simulink model "Lab2_Challenge"  (R2020b)
settings: Solver=VariableStepAuto  StartTime=0.0  StopTime=Time_of_simulation  RelTol=1e-3
undefined symbols (not defined in the file): A0, B0, Beq_hat, C, C0, D0, D_H_1, daq, degs2rpm, DiscIntNeverNeededParam, drv, Gamma_o, gbox, H, H_o, J_o, Jeq, K, K_I, Kw, Kw2, mot, N_H_1, Nr, Nu, Nx, Phi_o, rads2rpm, rpm2rads, sens, Step_ref, T, Ts
settings Model: Creator=Davide  LastModifiedBy=Musta

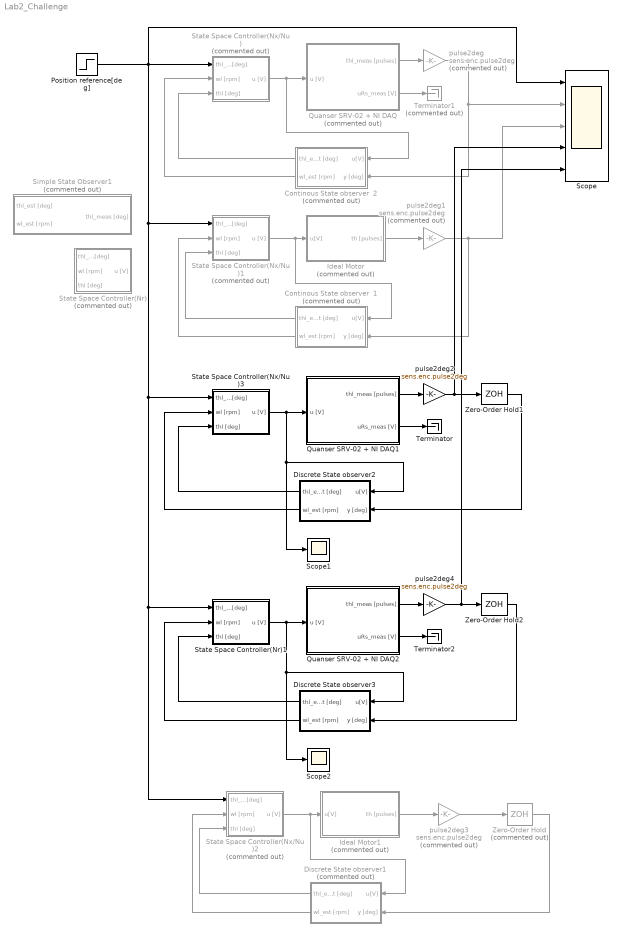
== system Lab2_Challenge ==
  Continous State observer  1 : Subsystem  Commented=on
  Continous State observer  2 : Subsystem  Commented=on
  Discrete State observer1 : Subsystem  Commented=on
  Discrete State observer2 : Subsystem
  Discrete State observer3 : Subsystem
  Ideal Motor : Subsystem  Commented=on
  Ideal Motor1 : Subsystem  Commented=on
  Position reference[deg] : Step  Time=0  After=Step_ref  SampleTime=0
  Quanser SRV-02 + NI DAQ : Subsystem  Commented=on  mask(Quanser SRV-02 (with inertial load) + NI DAQ){Ts=0.001, fricType=Coulomb + viscous}
      mask prompts: Ts "NI DAQ Sample Time:"; fricType "Friction model"
      mask help: Quanser SRV-02 (with inertial load) + NI DAQ model.
      mask init:
      | %%  Sensors data
      | 
      | %   shunt resistor
      | sens.curr.Rs = 0.5;                         %   resistance [Ohm]   
      | sens.curr.uRs_std = 0.01;                   %   voltage noise standard dev [V]                           
      | sens.curr.uRs_var = sens.curr.uRs_std^2;	%   voltage noise variance [V^2]
      | 
      | %   Hewlett-Packard HEDS-5540#A06 optical encoder
      | sens.enc.ppr = 500*4;                       %   pulses per rotation
      | sens.enc.pulse2deg = 360/sens.enc.ppr;      %   [pulses] -> [deg]
      | sens.enc.pulse2rad = 2*pi/sens.enc.ppr;     %   [pulses] -> [rad]
      | sens.enc.deg2pulse = sens.enc.ppr/360;      %   [deg] -> [pulses]
      | sens.enc.rad2pulse = sens.enc.ppr/2/pi;     %   [rad] -> [pulses]
      | 
      | 
      | %%  Data acquisition board (daq) data
      | 
      | %   NI PCI-6221 DAC data
      | daq.dac.bits = 16;                                  %   resolution (bits)
      | daq.dac.fs   = 10;                                  %   full scale 
      | daq.dac.q    = 2*daq.dac.fs/(2^daq.dac.bits-1);     %	quantization
      | 
      | %   NI PCI-6221 ADC data
      | daq.adc.bits = 16;                                  %   resolution (bits)
      | daq.adc.fs   = 10;                                  %   full scale (as set in SLDRT Analog Input block)
      | daq.adc.q    = 2*daq.adc.fs/(2^daq.adc.bits-1);     %   quantization
      mask Help:
      | Riccardo Antonello (antonello@dei.unipd.it)
      | 
      | April 24, 2020
      | 
      | Dept. of Information Engineering, University of Padova
      mask TypeOptions fricType: Coulomb + viscous | Karnopp
  Quanser SRV-02 + NI DAQ1 : Subsystem  mask(Quanser SRV-02 (with inertial load) + NI DAQ){Ts=T, fricType=Karnopp}
      mask prompts: Ts "NI DAQ Sample Time:"; fricType "Friction model"
      mask help: Quanser SRV-02 (with inertial load) + NI DAQ model.
      mask init: same as Lab2_Challenge/Quanser SRV-02 + NI DAQ
      mask Help:
      | Riccardo Antonello (antonello@dei.unipd.it)
      | 
      | April 24, 2020
      | 
      | Dept. of Information Engineering, University of Padova
      mask TypeOptions fricType: Coulomb + viscous | Karnopp
  Quanser SRV-02 + NI DAQ2 : Subsystem  mask(Quanser SRV-02 (with inertial load) + NI DAQ){Ts=T, fricType=Karnopp}
      mask prompts: Ts "NI DAQ Sample Time:"; fricType "Friction model"
      mask help: Quanser SRV-02 (with inertial load) + NI DAQ model.
      mask init: same as Lab2_Challenge/Quanser SRV-02 + NI DAQ
      mask Help:
      | Riccardo Antonello (antonello@dei.unipd.it)
      | 
      | April 24, 2020
      | 
      | Dept. of Information Engineering, University of Padova
      mask TypeOptions fricType: Coulomb + viscous | Karnopp
  Scope : Scope  NumInputPorts=5
  Scope1 : Scope
  Scope2 : Scope
  Simple State Observer1 : Subsystem  Commented=on
  State Space Controller(Nr) : Subsystem  Commented=on
  State Space Controller(Nr)1 : Subsystem
  State Space Controller(Nx/Nu) : Subsystem  Commented=on
  State Space Controller(Nx/Nu)1 : Subsystem  Commented=on
  State Space Controller(Nx/Nu)2 : Subsystem  Commented=on
  State Space Controller(Nx/Nu)3 : Subsystem
  Terminator : Terminator
  Terminator1 : Terminator  Commented=on
  Terminator2 : Terminator
  Zero-Order Hold : ZeroOrderHold  Commented=on  SampleTime=T
  Zero-Order Hold1 : ZeroOrderHold  SampleTime=T
  Zero-Order Hold2 : ZeroOrderHold  SampleTime=T
  pulse2deg : Gain  Commented=on  Gain=sens.enc.pulse2deg
  pulse2deg1 : Gain  Commented=on  Gain=sens.enc.pulse2deg
  pulse2deg2 : Gain  Gain=sens.enc.pulse2deg
  pulse2deg3 : Gain  Commented=on  Gain=sens.enc.pulse2deg
  pulse2deg4 : Gain  Gain=sens.enc.pulse2deg
  wires:
  Quanser SRV-02 + NI DAQ/1(thl_meas [pulses]) -> pulse2deg/1
  pulse2deg/1 -> Continous State observer  2/2(y [deg]), Scope/2
  Continous State observer  2/1(thl_est [deg]) -> State Space Controller(Nx/Nu)/3(thl [deg])
  Continous State observer  2/2(wl_est [rpm]) -> State Space Controller(Nx/Nu)/2(wl [rpm])
  State Space Controller(Nx/Nu)/1(u [V]) -> Continous State observer  2/1(u[V]), Quanser SRV-02 + NI DAQ/1(u [V])
  Continous State observer  1/1(thl_est [deg]) -> State Space Controller(Nx/Nu)1/3(thl [deg])
  Continous State observer  1/2(wl_est [rpm]) -> State Space Controller(Nx/Nu)1/2(wl [rpm])
  Ideal Motor/1(th [pulses]) -> pulse2deg1/1
  State Space Controller(Nx/Nu)1/1(u [V]) -> Continous State observer  1/1(u[V]), Ideal Motor/1(u[V])
  pulse2deg1/1 -> Continous State observer  1/2(y [deg]), Scope/3
  State Space Controller(Nx/Nu)2/1(u [V]) -> Discrete State observer1/1(u[V]), Ideal Motor1/1(u[V])
  Ideal Motor1/1(th [pulses]) -> pulse2deg3/1
  Discrete State observer1/2(wl_est [rpm]) -> State Space Controller(Nx/Nu)2/2(wl [rpm])
  Discrete State observer1/1(thl_est [deg]) -> State Space Controller(Nx/Nu)2/3(thl [deg])
  State Space Controller(Nx/Nu)3/1(u [V]) -> Scope1/1, Discrete State observer2/1(u[V]), Quanser SRV-02 + NI DAQ1/1(u [V])
  Discrete State observer2/2(wl_est [rpm]) -> State Space Controller(Nx/Nu)3/2(wl [rpm])
  Discrete State observer2/1(thl_est [deg]) -> State Space Controller(Nx/Nu)3/3(thl [deg])
  Quanser SRV-02 + NI DAQ1/1(thl_meas [pulses]) -> pulse2deg2/1
  pulse2deg3/1 -> Zero-Order Hold/1
  pulse2deg2/1 -> Scope/4, Zero-Order Hold1/1
  Quanser SRV-02 + NI DAQ1/2(uRs_meas [V]) -> Terminator/1
  Quanser SRV-02 + NI DAQ/2(uRs_meas [V]) -> Terminator1/1
  Zero-Order Hold/1 -> Discrete State observer1/2(y [deg])
  Zero-Order Hold2/1 -> Discrete State observer3/2(y [deg])
  Quanser SRV-02 + NI DAQ2/2(uRs_meas [V]) -> Terminator2/1
  pulse2deg4/1 -> Scope/5, Zero-Order Hold2/1
  Quanser SRV-02 + NI DAQ2/1(thl_meas [pulses]) -> pulse2deg4/1
  Discrete State observer3/1(thl_est [deg]) -> State Space Controller(Nr)1/3(thl [deg])
  Discrete State observer3/2(wl_est [rpm]) -> State Space Controller(Nr)1/2(wl [rpm])
  State Space Controller(Nr)1/1(u [V]) -> Quanser SRV-02 + NI DAQ2/1(u [V]), Discrete State observer3/1(u[V]), Scope2/1
  Position reference[deg]/1 -> State Space Controller(Nx/Nu)3/1(thl_ref [deg]), State Space Controller(Nr)1/1(thl_ref [deg]), State Space Controller(Nx/Nu)2/1(thl_ref [deg]), State Space Controller(Nx/Nu)1/1(thl_ref [deg]), Scope/1, State Space Controller(Nx/Nu)/1(thl_ref [deg])
  Zero-Order Hold1/1 -> Discrete State observer2/2(y [deg])

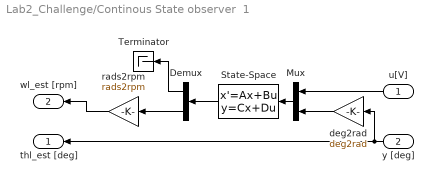
== system Lab2_Challenge/Continous State observer  1 ==
  u[V] : Inport
  y [deg] : Inport  Port=2
  Demux : Demux  Outputs=2
  Mux : Mux  Inputs=2
  State-Space : StateSpace  A=A0  B=B0  C=C0  D=D0  InitialCondition=0
  Terminator : Terminator
  deg2rad : Gain  Gain=deg2rad
  rads2rpm : Gain  Gain=rads2rpm
  thl_est [deg] : Outport
  wl_est [rpm] : Outport  Port=2
  wires:
  y [deg]/1 -> thl_est [deg]/1, deg2rad/1
  rads2rpm/1 -> wl_est [rpm]/1
  Demux/2 -> rads2rpm/1
  deg2rad/1 -> Mux/2
  State-Space/1 -> Demux/1
  Mux/1 -> State-Space/1
  u[V]/1 -> Mux/1
  Demux/1 -> Terminator/1

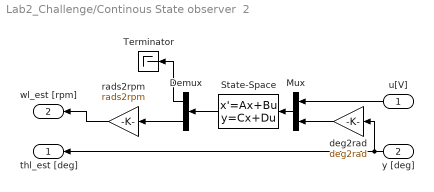
== system Lab2_Challenge/Continous State observer  2 ==
  u[V] : Inport
  y [deg] : Inport  Port=2
  Demux : Demux  Outputs=2
  Mux : Mux  Inputs=2
  State-Space : StateSpace  A=A0  B=B0  C=C0  D=D0  InitialCondition=0
  Terminator : Terminator
  deg2rad : Gain  Gain=deg2rad
  rads2rpm : Gain  Gain=rads2rpm
  thl_est [deg] : Outport
  wl_est [rpm] : Outport  Port=2
  wires:
  u[V]/1 -> Mux/1
  Mux/1 -> State-Space/1
  State-Space/1 -> Demux/1
  deg2rad/1 -> Mux/2
  Demux/2 -> rads2rpm/1
  rads2rpm/1 -> wl_est [rpm]/1
  y [deg]/1 -> deg2rad/1, thl_est [deg]/1
  Demux/1 -> Terminator/1

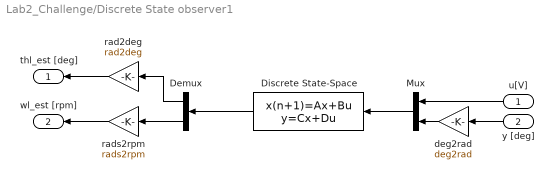
== system Lab2_Challenge/Discrete State observer1 ==
  u[V] : Inport
  y [deg] : Inport  Port=2
  Demux : Demux  Outputs=2
  Discrete State-Space : DiscreteStateSpace  A=Phi_o  B=Gamma_o  C=H_o  D=J_o  SampleTime=T
  Mux : Mux  Inputs=2
  deg2rad : Gain  Gain=deg2rad
  rad2deg : Gain  Gain=rad2deg
  rads2rpm : Gain  Gain=rads2rpm
  thl_est [deg] : Outport
  wl_est [rpm] : Outport  Port=2
  wires:
  Demux/1 -> rad2deg/1
  rad2deg/1 -> thl_est [deg]/1
  u[V]/1 -> Mux/1
  Mux/1 -> Discrete State-Space/1
  Discrete State-Space/1 -> Demux/1
  deg2rad/1 -> Mux/2
  Demux/2 -> rads2rpm/1
  rads2rpm/1 -> wl_est [rpm]/1
  y [deg]/1 -> deg2rad/1

== system Lab2_Challenge/Discrete State observer2 ==
  u[V] : Inport
  y [deg] : Inport  Port=2
  Demux : Demux  Outputs=2
  Discrete State-Space : DiscreteStateSpace  A=Phi_o  B=Gamma_o  C=H_o  D=J_o  SampleTime=T
  Mux : Mux  Inputs=2
  deg2rad : Gain  Gain=deg2rad
  rad2deg : Gain  Gain=rad2deg
  rads2rpm : Gain  Gain=rads2rpm
  thl_est [deg] : Outport
  wl_est [rpm] : Outport  Port=2
  wires:
  y [deg]/1 -> deg2rad/1
  rads2rpm/1 -> wl_est [rpm]/1
  Demux/2 -> rads2rpm/1
  deg2rad/1 -> Mux/2
  Discrete State-Space/1 -> Demux/1
  Mux/1 -> Discrete State-Space/1
  u[V]/1 -> Mux/1
  rad2deg/1 -> thl_est [deg]/1
  Demux/1 -> rad2deg/1

== system Lab2_Challenge/Discrete State observer3 ==
  u[V] : Inport
  y [deg] : Inport  Port=2
  Demux : Demux  Outputs=2
  Discrete State-Space : DiscreteStateSpace  A=Phi_o  B=Gamma_o  C=H_o  D=J_o  SampleTime=T
  Mux : Mux  Inputs=2
  deg2rad : Gain  Gain=deg2rad
  rad2deg : Gain  Gain=rad2deg
  rads2rpm : Gain  Gain=rads2rpm
  thl_est [deg] : Outport
  wl_est [rpm] : Outport  Port=2
  wires:
  Demux/1 -> rad2deg/1
  rad2deg/1 -> thl_est [deg]/1
  u[V]/1 -> Mux/1
  Mux/1 -> Discrete State-Space/1
  Discrete State-Space/1 -> Demux/1
  deg2rad/1 -> Mux/2
  Demux/2 -> rads2rpm/1
  rads2rpm/1 -> wl_est [rpm]/1
  y [deg]/1 -> deg2rad/1

== system Lab2_Challenge/Ideal Motor ==
  u[V] : Inport
  DAC : Subsystem
  DC motor + gearbox : Subsystem
  Enocder : Subsystem
  Voltage driver : Subsystem
  th [pulses] : Outport
  wires:
  Voltage driver/1(udrv[V]) -> DC motor + gearbox/1(udrv[V])  "udrv"
  DAC/1(Out) -> Voltage driver/1(u[V])
  u[V]/1 -> DAC/1(u[V])
  Enocder/1(th [pulses]) -> th [pulses]/1
  DC motor + gearbox/2(thl[deg]) -> Enocder/1(th [deg])  "thi_meas"

== system Lab2_Challenge/Ideal Motor1 ==
  u[V] : Inport
  DAC : Subsystem
  DC motor + gearbox : Subsystem
  Enocder : Subsystem
  Voltage driver : Subsystem
  th [pulses] : Outport
  wires:
  DC motor + gearbox/2(thl[deg]) -> Enocder/1(th [deg])  "thi_meas"
  Enocder/1(th [pulses]) -> th [pulses]/1
  u[V]/1 -> DAC/1(u[V])
  DAC/1(Out) -> Voltage driver/1(u[V])
  Voltage driver/1(udrv[V]) -> DC motor + gearbox/1(udrv[V])  "udrv"

== system Lab2_Challenge/Quanser SRV-02 + NI DAQ ==
  u [V] : Inport
  ADC : Subsystem
  Constant : Constant  Value=fricType
  DAC : Subsystem
  Enocder : Subsystem
  Quanser SRV-02 : ModelReference  ModelNameDialog=SRV02IL_win64.slxp  ModelReferenceVersion=1.44  CopyOfModelProtected=on
  Terminator1 : Terminator
  Terminator2 : Terminator
  thl_meas [pulses] : Outport
  uRs_meas [V] : Outport  Port=2
  wires:
  Enocder/1(th [pulses]) -> thl_meas [pulses]/1
  ADC/1(Out) -> uRs_meas [V]/1
  DAC/1(Out) -> Quanser SRV-02/1
  Quanser SRV-02/2 -> ADC/1(In), Terminator1/1
  u [V]/1 -> DAC/1(In)
  Quanser SRV-02/1 -> Enocder/1(th [deg]), Terminator2/1
  Constant/1 -> Quanser SRV-02/2

== system Lab2_Challenge/Quanser SRV-02 + NI DAQ1 ==
  u [V] : Inport
  ADC : Subsystem
  Constant : Constant  Value=fricType
  DAC : Subsystem
  Enocder : Subsystem
  Quanser SRV-02 : ModelReference  ModelNameDialog=SRV02IL_win64.slxp  ModelReferenceVersion=1.44  CopyOfModelProtected=on
  Terminator1 : Terminator
  Terminator2 : Terminator
  thl_meas [pulses] : Outport
  uRs_meas [V] : Outport  Port=2
  wires:
  Constant/1 -> Quanser SRV-02/2
  Quanser SRV-02/1 -> Terminator2/1, Enocder/1(th [deg])
  u [V]/1 -> DAC/1(In)
  Quanser SRV-02/2 -> Terminator1/1, ADC/1(In)
  DAC/1(Out) -> Quanser SRV-02/1
  ADC/1(Out) -> uRs_meas [V]/1
  Enocder/1(th [pulses]) -> thl_meas [pulses]/1

== system Lab2_Challenge/Quanser SRV-02 + NI DAQ2 ==
  u [V] : Inport
  ADC : Subsystem
  Constant : Constant  Value=fricType
  DAC : Subsystem
  Enocder : Subsystem
  Quanser SRV-02 : ModelReference  ModelNameDialog=SRV02IL_win64.slxp  ModelReferenceVersion=1.44  CopyOfModelProtected=on
  Terminator1 : Terminator
  Terminator2 : Terminator
  thl_meas [pulses] : Outport
  uRs_meas [V] : Outport  Port=2
  wires:
  Enocder/1(th [pulses]) -> thl_meas [pulses]/1
  ADC/1(Out) -> uRs_meas [V]/1
  DAC/1(Out) -> Quanser SRV-02/1
  Quanser SRV-02/2 -> ADC/1(In), Terminator1/1
  u [V]/1 -> DAC/1(In)
  Quanser SRV-02/1 -> Enocder/1(th [deg]), Terminator2/1
  Constant/1 -> Quanser SRV-02/2

== system Lab2_Challenge/Simple State Observer1 ==
  thl_meas [deg] : Inport
  Real derivative : TransferFcn  Numerator=[N_H_1]  Denominator=[D_H_1]
  degs2rpm : Gain  Gain=degs2rpm
  thl_est [deg] : Outport
  wl_est [rpm] : Outport  Port=2
  wires:
  degs2rpm/1 -> wl_est [rpm]/1
  thl_meas [deg]/1 -> Real derivative/1, thl_est [deg]/1
  Real derivative/1 -> degs2rpm/1

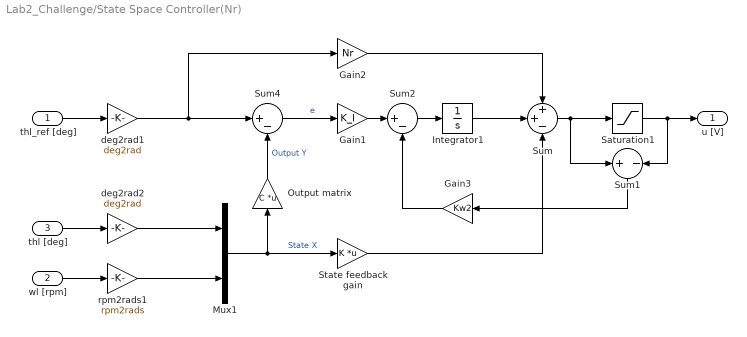
== system Lab2_Challenge/State Space Controller(Nr) ==
  thl_ref [deg] : Inport
  wl [rpm] : Inport  Port=2
  thl [deg] : Inport  Port=3
  Gain1 : Gain  Gain=K_I
  Gain2 : Gain  Gain=Nr
  Gain3 : Gain  Gain=Kw2
  Integrator1 : Integrator
  Mux1 : Mux  Inputs=2
  Output matrix : Gain  Gain=C  Multiplication=Matrix(K*u)
  Saturation1 : Saturate  UpperLimit=daq.dac.fs  LowerLimit=-daq.dac.fs
  State feedback gain : Gain  Gain=K  Multiplication=Matrix(K*u)
  Sum : Sum  Inputs=++-
  Sum1 : Sum  Inputs=+|-
  Sum2 : Sum  Inputs=|+-
  Sum4 : Sum  Inputs=|+-
  deg2rad1 : Gain  Gain=deg2rad
  deg2rad2 : Gain  Gain=deg2rad
  rpm2rads1 : Gain  Gain=rpm2rads
  u [V] : Outport
  wires:
  thl [deg]/1 -> deg2rad2/1
  wl [rpm]/1 -> rpm2rads1/1
  rpm2rads1/1 -> Mux1/2
  deg2rad2/1 -> Mux1/1
  thl_ref [deg]/1 -> deg2rad1/1
  Mux1/1 -> State feedback gain/1, Output matrix/1  "State X"
  State feedback gain/1 -> Sum/3
  Gain2/1 -> Sum/1
  Integrator1/1 -> Sum/2
  deg2rad1/1 -> Gain2/1, Sum4/1
  Output matrix/1 -> Sum4/2  "Output Y"
  Gain1/1 -> Sum2/1
  Sum4/1 -> Gain1/1  "e"
  Gain3/1 -> Sum2/2
  Sum1/1 -> Gain3/1
  Sum2/1 -> Integrator1/1
  Saturation1/1 -> u [V]/1, Sum1/2
  Sum/1 -> Saturation1/1, Sum1/1

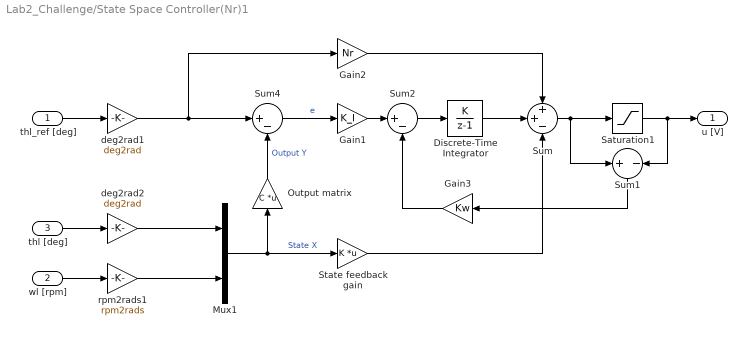
== system Lab2_Challenge/State Space Controller(Nr)1 ==
  thl_ref [deg] : Inport
  wl [rpm] : Inport  Port=2
  thl [deg] : Inport  Port=3
  Discrete-Time Integrator : DiscreteIntegrator  IntegratorMethod=Accumulation: Forward Euler  SampleTime=T  ICPrevOutput=DiscIntNeverNeededParam  ICPrevScaledInput=DiscIntNeverNeededParam
  Gain1 : Gain  Gain=K_I
  Gain2 : Gain  Gain=Nr
  Gain3 : Gain  Gain=Kw
  Mux1 : Mux  Inputs=2
  Output matrix : Gain  Gain=C  Multiplication=Matrix(K*u)
  Saturation1 : Saturate  UpperLimit=daq.dac.fs  LowerLimit=-daq.dac.fs
  State feedback gain : Gain  Gain=K  Multiplication=Matrix(K*u)
  Sum : Sum  Inputs=++-
  Sum1 : Sum  Inputs=+|-
  Sum2 : Sum  Inputs=|+-
  Sum4 : Sum  Inputs=|+-
  deg2rad1 : Gain  Gain=deg2rad
  deg2rad2 : Gain  Gain=deg2rad
  rpm2rads1 : Gain  Gain=rpm2rads
  u [V] : Outport
  wires:
  thl [deg]/1 -> deg2rad2/1
  wl [rpm]/1 -> rpm2rads1/1
  rpm2rads1/1 -> Mux1/2
  deg2rad2/1 -> Mux1/1
  thl_ref [deg]/1 -> deg2rad1/1
  Mux1/1 -> State feedback gain/1, Output matrix/1  "State X"
  State feedback gain/1 -> Sum/3
  Gain2/1 -> Sum/1
  Discrete-Time Integrator/1 -> Sum/2
  deg2rad1/1 -> Gain2/1, Sum4/1
  Output matrix/1 -> Sum4/2  "Output Y"
  Gain1/1 -> Sum2/1
  Sum4/1 -> Gain1/1  "e"
  Gain3/1 -> Sum2/2
  Sum1/1 -> Gain3/1
  Sum2/1 -> Discrete-Time Integrator/1
  Saturation1/1 -> u [V]/1, Sum1/2
  Sum/1 -> Saturation1/1, Sum1/1

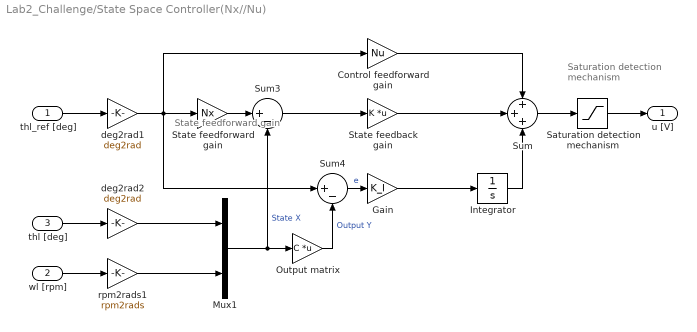
== system Lab2_Challenge/State Space Controller(Nx//Nu) ==
  note: State feedforward
      | gain
  note: Saturation
      | detection
      | mechanism
  thl_ref [deg] : Inport
  wl [rpm] : Inport  Port=2
  thl [deg] : Inport  Port=3
  Control feedforward gain : Gain  Gain=Nu
  Gain : Gain  Gain=K_I
  Integrator : Integrator
  Mux1 : Mux  Inputs=2
  Output matrix : Gain  Gain=C  Multiplication=Matrix(K*u)
  Saturation detection mechanism : Saturate  UpperLimit=daq.dac.fs  LowerLimit=-daq.dac.fs
  State feedback gain : Gain  Gain=K  Multiplication=Matrix(K*u)
  State feedforward gain : Gain  Gain=Nx
  Sum : Sum  Inputs=+++
  Sum3 : Sum  Inputs=|+-
  Sum4 : Sum  Inputs=|+-
  deg2rad1 : Gain  Gain=deg2rad
  deg2rad2 : Gain  Gain=deg2rad
  rpm2rads1 : Gain  Gain=rpm2rads
  u [V] : Outport
  wires:
  thl [deg]/1 -> deg2rad2/1
  wl [rpm]/1 -> rpm2rads1/1
  Sum/1 -> Saturation detection mechanism/1
  Saturation detection mechanism/1 -> u [V]/1
  rpm2rads1/1 -> Mux1/2
  deg2rad2/1 -> Mux1/1
  thl_ref [deg]/1 -> deg2rad1/1
  State feedforward gain/1 -> Sum3/1
  Mux1/1 -> Output matrix/1, Sum3/2  "State X"
  Sum3/1 -> State feedback gain/1
  State feedback gain/1 -> Sum/2
  Control feedforward gain/1 -> Sum/1
  Output matrix/1 -> Sum4/2  "Output Y"
  deg2rad1/1 -> State feedforward gain/1, Sum4/1, Control feedforward gain/1
  Gain/1 -> Integrator/1
  Sum4/1 -> Gain/1  "e"
  Integrator/1 -> Sum/3

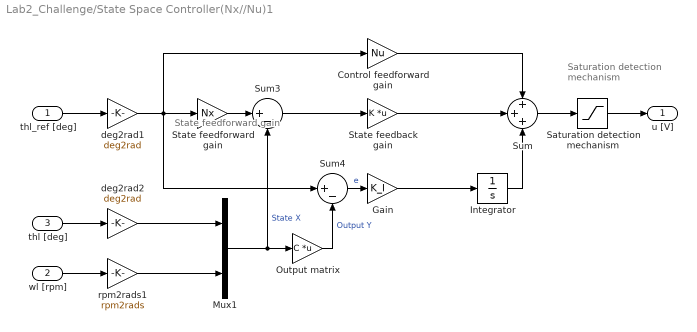
== system Lab2_Challenge/State Space Controller(Nx//Nu)1 ==
  note: Saturation
      | detection
      | mechanism
  note: State feedforward
      | gain
  thl_ref [deg] : Inport
  wl [rpm] : Inport  Port=2
  thl [deg] : Inport  Port=3
  Control feedforward gain : Gain  Gain=Nu
  Gain : Gain  Gain=K_I
  Integrator : Integrator
  Mux1 : Mux  Inputs=2
  Output matrix : Gain  Gain=C  Multiplication=Matrix(K*u)
  Saturation detection mechanism : Saturate  UpperLimit=daq.dac.fs  LowerLimit=-daq.dac.fs
  State feedback gain : Gain  Gain=K  Multiplication=Matrix(K*u)
  State feedforward gain : Gain  Gain=Nx
  Sum : Sum  Inputs=+++
  Sum3 : Sum  Inputs=|+-
  Sum4 : Sum  Inputs=|+-
  deg2rad1 : Gain  Gain=deg2rad
  deg2rad2 : Gain  Gain=deg2rad
  rpm2rads1 : Gain  Gain=rpm2rads
  u [V] : Outport
  wires:
  Integrator/1 -> Sum/3
  Sum4/1 -> Gain/1  "e"
  Gain/1 -> Integrator/1
  deg2rad1/1 -> Control feedforward gain/1, Sum4/1, State feedforward gain/1
  Output matrix/1 -> Sum4/2  "Output Y"
  Control feedforward gain/1 -> Sum/1
  State feedback gain/1 -> Sum/2
  Sum3/1 -> State feedback gain/1
  Mux1/1 -> Sum3/2, Output matrix/1  "State X"
  State feedforward gain/1 -> Sum3/1
  thl_ref [deg]/1 -> deg2rad1/1
  deg2rad2/1 -> Mux1/1
  rpm2rads1/1 -> Mux1/2
  Saturation detection mechanism/1 -> u [V]/1
  Sum/1 -> Saturation detection mechanism/1
  wl [rpm]/1 -> rpm2rads1/1
  thl [deg]/1 -> deg2rad2/1

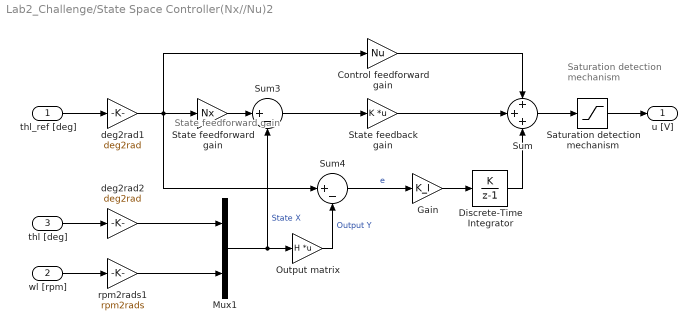
== system Lab2_Challenge/State Space Controller(Nx//Nu)2 ==
  note: Saturation
      | detection
      | mechanism
  note: State feedforward
      | gain
  thl_ref [deg] : Inport
  wl [rpm] : Inport  Port=2
  thl [deg] : Inport  Port=3
  Control feedforward gain : Gain  Gain=Nu
  Discrete-Time Integrator : DiscreteIntegrator  IntegratorMethod=Accumulation: Forward Euler  SampleTime=T  ICPrevOutput=DiscIntNeverNeededParam  ICPrevScaledInput=DiscIntNeverNeededParam
  Gain : Gain  Gain=K_I
  Mux1 : Mux  Inputs=2
  Output matrix : Gain  Gain=H  Multiplication=Matrix(K*u)
  Saturation detection mechanism : Saturate  UpperLimit=daq.dac.fs  LowerLimit=-daq.dac.fs
  State feedback gain : Gain  Gain=K  Multiplication=Matrix(K*u)
  State feedforward gain : Gain  Gain=Nx
  Sum : Sum  Inputs=+++
  Sum3 : Sum  Inputs=|+-
  Sum4 : Sum  Inputs=|+-
  deg2rad1 : Gain  Gain=deg2rad
  deg2rad2 : Gain  Gain=deg2rad
  rpm2rads1 : Gain  Gain=rpm2rads
  u [V] : Outport
  wires:
  Discrete-Time Integrator/1 -> Sum/3
  Sum4/1 -> Gain/1  "e"
  Gain/1 -> Discrete-Time Integrator/1
  deg2rad1/1 -> Control feedforward gain/1, Sum4/1, State feedforward gain/1
  Output matrix/1 -> Sum4/2  "Output Y"
  Control feedforward gain/1 -> Sum/1
  State feedback gain/1 -> Sum/2
  Sum3/1 -> State feedback gain/1
  Mux1/1 -> Sum3/2, Output matrix/1  "State X"
  State feedforward gain/1 -> Sum3/1
  thl_ref [deg]/1 -> deg2rad1/1
  deg2rad2/1 -> Mux1/1
  rpm2rads1/1 -> Mux1/2
  Saturation detection mechanism/1 -> u [V]/1
  Sum/1 -> Saturation detection mechanism/1
  wl [rpm]/1 -> rpm2rads1/1
  thl [deg]/1 -> deg2rad2/1

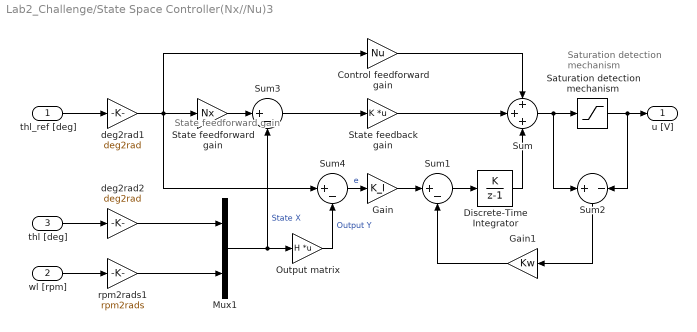
== system Lab2_Challenge/State Space Controller(Nx//Nu)3 ==
  note: State feedforward
      | gain
  note: Saturation
      | detection
      | mechanism
  thl_ref [deg] : Inport
  wl [rpm] : Inport  Port=2
  thl [deg] : Inport  Port=3
  Control feedforward gain : Gain  Gain=Nu
  Discrete-Time Integrator : DiscreteIntegrator  IntegratorMethod=Accumulation: Forward Euler  SampleTime=T  ICPrevOutput=DiscIntNeverNeededParam  ICPrevScaledInput=DiscIntNeverNeededParam
  Gain : Gain  Gain=K_I
  Gain1 : Gain  Gain=Kw
  Mux1 : Mux  Inputs=2
  Output matrix : Gain  Gain=H  Multiplication=Matrix(K*u)
  Saturation detection mechanism : Saturate  UpperLimit=daq.dac.fs  LowerLimit=-daq.dac.fs
  State feedback gain : Gain  Gain=K  Multiplication=Matrix(K*u)
  State feedforward gain : Gain  Gain=Nx
  Sum : Sum  Inputs=+++
  Sum1 : Sum  Inputs=|+-
  Sum2 : Sum  Inputs=+|-
  Sum3 : Sum  Inputs=|+-
  Sum4 : Sum  Inputs=|+-
  deg2rad1 : Gain  Gain=deg2rad
  deg2rad2 : Gain  Gain=deg2rad
  rpm2rads1 : Gain  Gain=rpm2rads
  u [V] : Outport
  wires:
  thl [deg]/1 -> deg2rad2/1
  wl [rpm]/1 -> rpm2rads1/1
  Sum/1 -> Sum2/1, Saturation detection mechanism/1
  Saturation detection mechanism/1 -> Sum2/2, u [V]/1
  rpm2rads1/1 -> Mux1/2
  deg2rad2/1 -> Mux1/1
  thl_ref [deg]/1 -> deg2rad1/1
  State feedforward gain/1 -> Sum3/1
  Mux1/1 -> Output matrix/1, Sum3/2  "State X"
  Sum3/1 -> State feedback gain/1
  State feedback gain/1 -> Sum/2
  Control feedforward gain/1 -> Sum/1
  Output matrix/1 -> Sum4/2  "Output Y"
  deg2rad1/1 -> State feedforward gain/1, Sum4/1, Control feedforward gain/1
  Gain/1 -> Sum1/1
  Sum4/1 -> Gain/1  "e"
  Discrete-Time Integrator/1 -> Sum/3
  Sum1/1 -> Discrete-Time Integrator/1
  Gain1/1 -> Sum1/2
  Sum2/1 -> Gain1/1

== system Lab2_Challenge/Ideal Motor/DAC ==
  u[V] : Inport
  Quantizer : Quantizer  QuantizationInterval=daq.dac.q
  Saturation : Saturate  UpperLimit=daq.dac.fs  LowerLimit=-daq.dac.fs
  Zero-Order Hold : ZeroOrderHold  SampleTime=Ts
  Out : Outport
  wires:
  Saturation/1 -> Out/1
  Zero-Order Hold/1 -> Quantizer/1
  u[V]/1 -> Zero-Order Hold/1
  Quantizer/1 -> Saturation/1

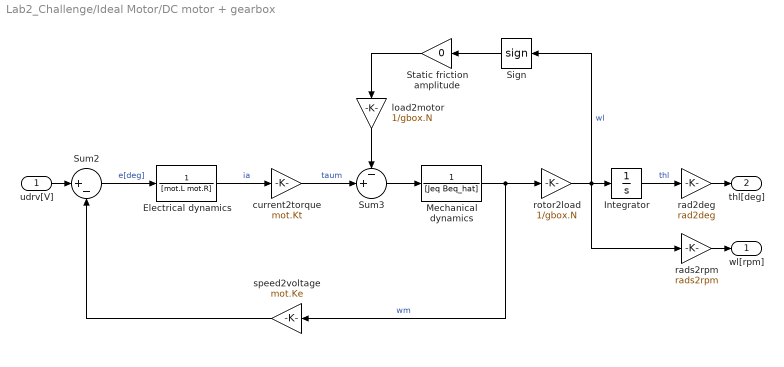
== system Lab2_Challenge/Ideal Motor/DC motor + gearbox ==
  udrv[V] : Inport
  Electrical dynamics : TransferFcn  Denominator=[mot.L mot.R]
  Integrator : Integrator
  Mechanical dynamics : TransferFcn  Denominator=[Jeq Beq_hat]
  Sign : Signum
  Static friction amplitude : Gain  Gain=0
  Sum2 : Sum  Inputs=|+-
  Sum3 : Sum  Inputs=-+|
  current2torque : Gain  Gain=mot.Kt
  load2motor : Gain  Gain=1/gbox.N
  rad2deg : Gain  Gain=rad2deg
  rads2rpm : Gain  Gain=rads2rpm
  rotor2load : Gain  Gain=1/gbox.N
  speed2voltage : Gain  Gain=mot.Ke
  wl[rpm] : Outport
  thl[deg] : Outport  Port=2
  wires:
  rotor2load/1 -> Sign/1, Integrator/1, rads2rpm/1  "wl"
  speed2voltage/1 -> Sum2/2
  load2motor/1 -> Sum3/1
  Sum3/1 -> Mechanical dynamics/1
  current2torque/1 -> Sum3/2  "taum"
  Static friction amplitude/1 -> load2motor/1
  Integrator/1 -> rad2deg/1  "thl"
  Electrical dynamics/1 -> current2torque/1  "ia"
  Sum2/1 -> Electrical dynamics/1  "e[deg]"
  Sign/1 -> Static friction amplitude/1
  rad2deg/1 -> thl[deg]/1
  Mechanical dynamics/1 -> speed2voltage/1, rotor2load/1  "wm"
  udrv[V]/1 -> Sum2/1
  rads2rpm/1 -> wl[rpm]/1

== system Lab2_Challenge/Ideal Motor/Enocder ==
  th [deg] : Inport
  Quantizer : Quantizer  QuantizationInterval=sens.enc.pulse2deg
  Zero-Order Hold : ZeroOrderHold  SampleTime=Ts
  deg2pulse : Gain  Gain=sens.enc.deg2pulse
  th [pulses] : Outport
  wires:
  deg2pulse/1 -> th [pulses]/1
  Zero-Order Hold/1 -> Quantizer/1
  th [deg]/1 -> Zero-Order Hold/1
  Quantizer/1 -> deg2pulse/1

== system Lab2_Challenge/Ideal Motor/Voltage driver ==
  u[V] : Inport
  Driver dynamics : TransferFcn  Numerator=[drv.dcgain]  Denominator=[drv.Tc 1]
  Driver saturation : Saturate  UpperLimit=drv.outmax  LowerLimit=-drv.outmax
  udrv[V] : Outport
  wires:
  Driver dynamics/1 -> Driver saturation/1
  u[V]/1 -> Driver dynamics/1
  Driver saturation/1 -> udrv[V]/1

== system Lab2_Challenge/Ideal Motor1/DAC ==
  u[V] : Inport
  Quantizer : Quantizer  QuantizationInterval=daq.dac.q
  Saturation : Saturate  UpperLimit=daq.dac.fs  LowerLimit=-daq.dac.fs
  Zero-Order Hold : ZeroOrderHold  SampleTime=Ts
  Out : Outport
  wires:
  Quantizer/1 -> Saturation/1
  u[V]/1 -> Zero-Order Hold/1
  Zero-Order Hold/1 -> Quantizer/1
  Saturation/1 -> Out/1

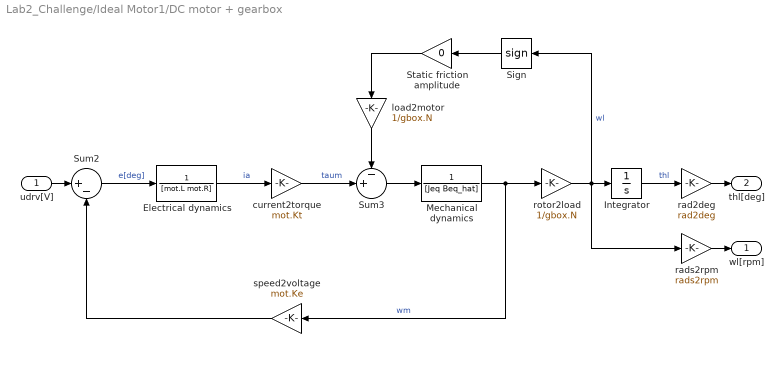
== system Lab2_Challenge/Ideal Motor1/DC motor + gearbox ==
  udrv[V] : Inport
  Electrical dynamics : TransferFcn  Denominator=[mot.L mot.R]
  Integrator : Integrator
  Mechanical dynamics : TransferFcn  Denominator=[Jeq Beq_hat]
  Sign : Signum
  Static friction amplitude : Gain  Gain=0
  Sum2 : Sum  Inputs=|+-
  Sum3 : Sum  Inputs=-+|
  current2torque : Gain  Gain=mot.Kt
  load2motor : Gain  Gain=1/gbox.N
  rad2deg : Gain  Gain=rad2deg
  rads2rpm : Gain  Gain=rads2rpm
  rotor2load : Gain  Gain=1/gbox.N
  speed2voltage : Gain  Gain=mot.Ke
  wl[rpm] : Outport
  thl[deg] : Outport  Port=2
  wires:
  rads2rpm/1 -> wl[rpm]/1
  udrv[V]/1 -> Sum2/1
  Mechanical dynamics/1 -> rotor2load/1, speed2voltage/1  "wm"
  rad2deg/1 -> thl[deg]/1
  Sign/1 -> Static friction amplitude/1
  Sum2/1 -> Electrical dynamics/1  "e[deg]"
  Electrical dynamics/1 -> current2torque/1  "ia"
  Integrator/1 -> rad2deg/1  "thl"
  Static friction amplitude/1 -> load2motor/1
  current2torque/1 -> Sum3/2  "taum"
  Sum3/1 -> Mechanical dynamics/1
  load2motor/1 -> Sum3/1
  speed2voltage/1 -> Sum2/2
  rotor2load/1 -> rads2rpm/1, Integrator/1, Sign/1  "wl"

== system Lab2_Challenge/Ideal Motor1/Enocder ==
  th [deg] : Inport
  Quantizer : Quantizer  QuantizationInterval=sens.enc.pulse2deg
  Zero-Order Hold : ZeroOrderHold  SampleTime=Ts
  deg2pulse : Gain  Gain=sens.enc.deg2pulse
  th [pulses] : Outport
  wires:
  Quantizer/1 -> deg2pulse/1
  th [deg]/1 -> Zero-Order Hold/1
  Zero-Order Hold/1 -> Quantizer/1
  deg2pulse/1 -> th [pulses]/1

== system Lab2_Challenge/Ideal Motor1/Voltage driver ==
  u[V] : Inport
  Driver dynamics : TransferFcn  Numerator=[drv.dcgain]  Denominator=[drv.Tc 1]
  Driver saturation : Saturate  UpperLimit=drv.outmax  LowerLimit=-drv.outmax
  udrv[V] : Outport
  wires:
  Driver saturation/1 -> udrv[V]/1
  u[V]/1 -> Driver dynamics/1
  Driver dynamics/1 -> Driver saturation/1

== system Lab2_Challenge/Quanser SRV-02 + NI DAQ/ADC ==
  In : Inport
  Quantizer : Quantizer  QuantizationInterval=daq.adc.q
  Saturation : Saturate  UpperLimit=daq.adc.fs  LowerLimit=-daq.adc.fs
  Zero-Order Hold : ZeroOrderHold  SampleTime=Ts
  Out : Outport
  wires:
  Saturation/1 -> Out/1
  In/1 -> Zero-Order Hold/1
  Quantizer/1 -> Saturation/1
  Zero-Order Hold/1 -> Quantizer/1

== system Lab2_Challenge/Quanser SRV-02 + NI DAQ/DAC ==
  In : Inport
  Quantizer : Quantizer  QuantizationInterval=daq.dac.q
  Saturation : Saturate  UpperLimit=daq.dac.fs  LowerLimit=-daq.dac.fs
  Zero-Order Hold : ZeroOrderHold  SampleTime=Ts
  Out : Outport
  wires:
  Quantizer/1 -> Saturation/1
  In/1 -> Zero-Order Hold/1
  Zero-Order Hold/1 -> Quantizer/1
  Saturation/1 -> Out/1

== system Lab2_Challenge/Quanser SRV-02 + NI DAQ/Enocder ==
  th [deg] : Inport
  Quantizer : Quantizer  QuantizationInterval=sens.enc.pulse2deg
  Zero-Order Hold : ZeroOrderHold  SampleTime=Ts
  deg2pulse : Gain  Gain=sens.enc.deg2pulse
  th [pulses] : Outport
  wires:
  Quantizer/1 -> deg2pulse/1
  th [deg]/1 -> Zero-Order Hold/1
  Zero-Order Hold/1 -> Quantizer/1
  deg2pulse/1 -> th [pulses]/1

== system Lab2_Challenge/Quanser SRV-02 + NI DAQ1/ADC ==
  In : Inport
  Quantizer : Quantizer  QuantizationInterval=daq.adc.q
  Saturation : Saturate  UpperLimit=daq.adc.fs  LowerLimit=-daq.adc.fs
  Zero-Order Hold : ZeroOrderHold  SampleTime=Ts
  Out : Outport
  wires:
  Zero-Order Hold/1 -> Quantizer/1
  Quantizer/1 -> Saturation/1
  In/1 -> Zero-Order Hold/1
  Saturation/1 -> Out/1

== system Lab2_Challenge/Quanser SRV-02 + NI DAQ1/DAC ==
  In : Inport
  Quantizer : Quantizer  QuantizationInterval=daq.dac.q
  Saturation : Saturate  UpperLimit=daq.dac.fs  LowerLimit=-daq.dac.fs
  Zero-Order Hold : ZeroOrderHold  SampleTime=Ts
  Out : Outport
  wires:
  Saturation/1 -> Out/1
  Zero-Order Hold/1 -> Quantizer/1
  In/1 -> Zero-Order Hold/1
  Quantizer/1 -> Saturation/1

== system Lab2_Challenge/Quanser SRV-02 + NI DAQ1/Enocder ==
  th [deg] : Inport
  Quantizer : Quantizer  QuantizationInterval=sens.enc.pulse2deg
  Zero-Order Hold : ZeroOrderHold  SampleTime=Ts
  deg2pulse : Gain  Gain=sens.enc.deg2pulse
  th [pulses] : Outport
  wires:
  deg2pulse/1 -> th [pulses]/1
  Zero-Order Hold/1 -> Quantizer/1
  th [deg]/1 -> Zero-Order Hold/1
  Quantizer/1 -> deg2pulse/1

== system Lab2_Challenge/Quanser SRV-02 + NI DAQ2/ADC ==
  In : Inport
  Quantizer : Quantizer  QuantizationInterval=daq.adc.q
  Saturation : Saturate  UpperLimit=daq.adc.fs  LowerLimit=-daq.adc.fs
  Zero-Order Hold : ZeroOrderHold  SampleTime=Ts
  Out : Outport
  wires:
  Saturation/1 -> Out/1
  In/1 -> Zero-Order Hold/1
  Quantizer/1 -> Saturation/1
  Zero-Order Hold/1 -> Quantizer/1

== system Lab2_Challenge/Quanser SRV-02 + NI DAQ2/DAC ==
  In : Inport
  Quantizer : Quantizer  QuantizationInterval=daq.dac.q
  Saturation : Saturate  UpperLimit=daq.dac.fs  LowerLimit=-daq.dac.fs
  Zero-Order Hold : ZeroOrderHold  SampleTime=Ts
  Out : Outport
  wires:
  Quantizer/1 -> Saturation/1
  In/1 -> Zero-Order Hold/1
  Zero-Order Hold/1 -> Quantizer/1
  Saturation/1 -> Out/1

== system Lab2_Challenge/Quanser SRV-02 + NI DAQ2/Enocder ==
  th [deg] : Inport
  Quantizer : Quantizer  QuantizationInterval=sens.enc.pulse2deg
  Zero-Order Hold : ZeroOrderHold  SampleTime=Ts
  deg2pulse : Gain  Gain=sens.enc.deg2pulse
  th [pulses] : Outport
  wires:
  Quantizer/1 -> deg2pulse/1
  th [deg]/1 -> Zero-Order Hold/1
  Zero-Order Hold/1 -> Quantizer/1
  deg2pulse/1 -> th [pulses]/1
